simulink model "modelOptim"  (Simulink 7.4)
settings: Solver=ode45  StartTime=0.0  StopTime=10.0  FixedStep=0.0056  RelTol=1e-3
values from neighbouring files (symbols this model uses):
  ad = Td/(Td + N*T0)    (= 0.994807351258)    [model_params.m]
  b = 0.2352    [model_params.m]
  bd = Kp*Td*N/(Td + N*T0)    (= 0.312545231066)    [model_params.m]
  bi1 = Kp*T0/Ti    (= 0.0654877697842)    [model_params.m]
  c = 0.7181    [model_params.m]
  Kp = K1(2:4)    [dlqr_reg.m]    (also in model_params.m = 0.6502)
  m = armax(datae,[3 3 3 1])    [dlqr_reg.m]    (also in model_params.m)
settings Model: Creator=Alex  LastModifiedBy=Alex
settings DebuggingCC: AlgebraicLoopMsg=none  ArtificialAlgebraicLoopMsg=none  SolverPrmCheckMsg=none  InheritedTsInSrcMsg=none  DiscreteInheritContinuousMsg=none  MultiTaskCondExecSysMsg=none  TasksWithSamePriorityMsg=none  SigSpecEnsureSampleTimeMsg=none  UnknownTsInhSupMsg=none  ModelReferenceExtraNoncontSigs=none  StateNameClashWarn=none  SimStateInterfaceChecksumMismatchMsg=none

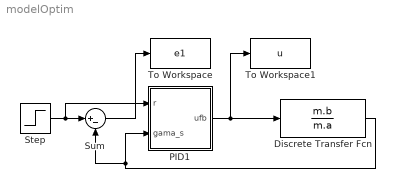
== system modelOptim ==
  Discrete Transfer Fcn : DiscreteTransferFcn  Numerator=m.b  Denominator=m.a  SampleTime=0.0056
  PID1 : Subsystem
  Step : Step  Time=0  After=0.1  SampleTime=0.0056  ZeroCross=off
  Sum : Sum  Inputs=|+-  OutDataType=fixdt(1, 16)  OutScaling=2^0
  To Workspace : ToWorkspace  VariableName=e1  SampleTime=-1  SaveFormat=Array
  To Workspace1 : ToWorkspace  VariableName=u  SampleTime=-1  SaveFormat=Array
  wires:
  PID1/1(ufb) -> Discrete Transfer Fcn/1, To Workspace1/1
  Discrete Transfer Fcn/1 -> PID1/2(gama_s), Sum/2
  Step/1 -> Sum/1, PID1/1(r)
  Sum/1 -> To Workspace/1

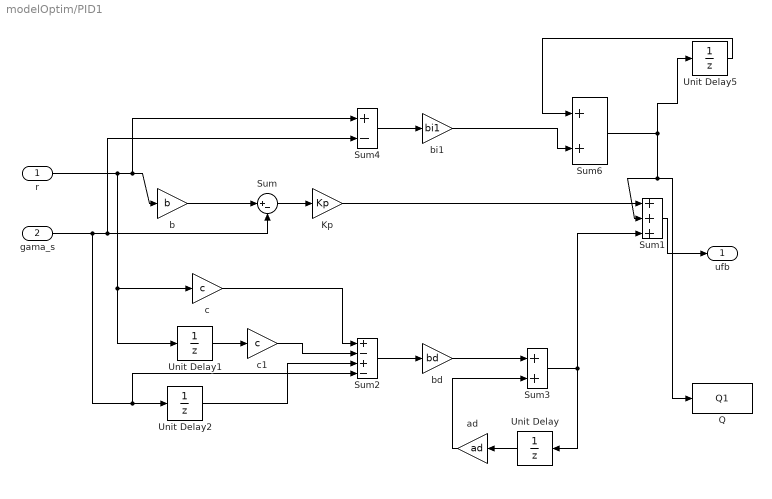
== system modelOptim/PID1 ==
  r : Inport
  gama_s : Inport  Port=2
  Kp : Gain  Gain=Kp
  Q : ToWorkspace  VariableName=Q1  SampleTime=-1  SaveFormat=Array
  Sum : Sum  Inputs=|+-
  Sum1 : Sum  Inputs=+++
  Sum2 : Sum  Inputs=+-+-
  Sum3 : Sum
  Sum4 : Sum  Inputs=+-
  Sum6 : Sum
  Unit Delay{,1..2,5} (4 alike) : UnitDelay  SampleTime=-1
  ad : Gain  Gain=ad
  b : Gain  Gain=b
  bd : Gain  Gain=bd
  bi1 : Gain  Gain=bi1
  c : Gain  Gain=c
  c1 : Gain  Gain=c
  ufb : Outport
  wires:
  Sum6/1 -> Unit Delay5/1, Q/1, Sum1/2
  bi1/1 -> Sum6/2
  Sum4/1 -> bi1/1
  Kp/1 -> Sum1/1
  Sum1/1 -> ufb/1
  Sum3/1 -> Sum1/3, Unit Delay/1
  bd/1 -> Sum3/1
  ad/1 -> Sum3/2
  Sum2/1 -> bd/1
  c1/1 -> Sum2/2
  c/1 -> Sum2/1
  Unit Delay2/1 -> Sum2/3
  Unit Delay1/1 -> c1/1
  Unit Delay/1 -> ad/1
  Sum/1 -> Kp/1
  gama_s/1 -> Sum/2, Sum4/2, Sum2/4, Unit Delay2/1
  b/1 -> Sum/1
  r/1 -> Sum4/1, b/1, Unit Delay1/1, c/1
  Unit Delay5/1 -> Sum6/1
